simulink model "Subsystem"  (R2020a)
settings: Solver=VariableStepAuto  StartTime=0.0  StopTime=10.0  RelTol=1e-3
model workspace (MAT data in the model file):
  J = Simulink.Parameter
  J.Value = 80
  J.DataType = 'auto'
  J.Dimensions = [1 1]
  K = Simulink.Parameter
  K.Value = 200
  K.DataType = 'auto'
  K.Dimensions = [1 1]
  L = Simulink.Parameter
  L.Value = 60
  L.DataType = 'auto'
  L.Dimensions = [1 1]
  R = Simulink.Parameter
  R.Value = 30
  R.DataType = 'auto'
  R.Dimensions = [1 1]
  b = Simulink.Parameter
  b.Value = 50
  b.DataType = 'auto'
  b.Dimensions = [1 1]
settings Model: Creator=anjal  LastModifiedBy=anjal
settings DataIOCC: SaveOutput=off  SaveTime=off

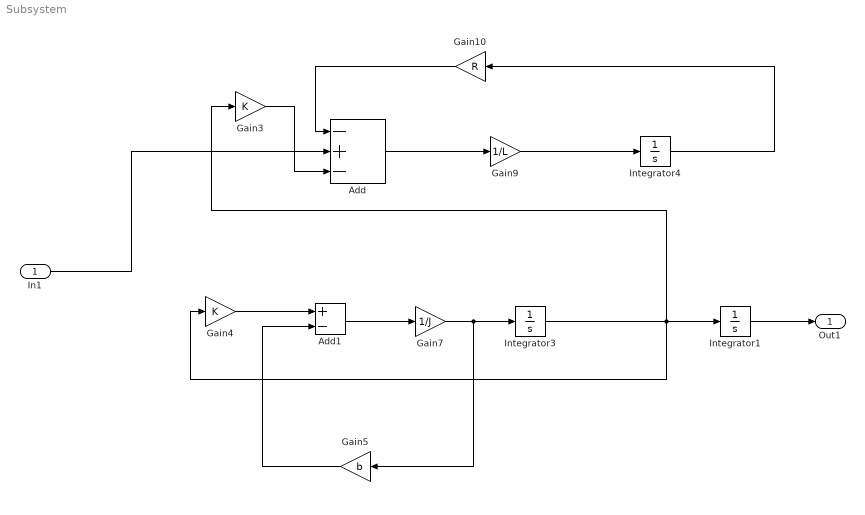
== system Subsystem ==
  In1 : Inport  OutDataTypeStr=double  PortDimensions=1  SampleTime=0
  Add : Sum  Inputs=-+-
  Add1 : Sum  Inputs=+-
  Gain10 : Gain  Gain=R
  Gain3 : Gain  Gain=K
  Gain4 : Gain  Gain=K
  Gain5 : Gain  Gain=b
  Gain7 : Gain  Gain=1/J
  Gain9 : Gain  Gain=1/L
  Integrator1 : Integrator
  Integrator3 : Integrator
  Integrator4 : Integrator
  Out1 : Outport  OutDataTypeStr=double  PortDimensions=1  SampleTime=0
  wires:
  Gain7/1 -> Integrator3/1, Gain5/1
  Gain4/1 -> Add1/1
  Gain5/1 -> Add1/2
  Integrator3/1 -> Gain4/1, Gain3/1, Integrator1/1
  Gain3/1 -> Add/3
  Gain9/1 -> Integrator4/1
  Integrator4/1 -> Gain10/1
  Add1/1 -> Gain7/1
  In1/1 -> Add/2
  Gain10/1 -> Add/1
  Add/1 -> Gain9/1
  Integrator1/1 -> Out1/1
